simulink library "Local_Lib"  (R2023a)
settings: Solver=VariableStepAuto  StartTime=0.0  StopTime=10.0  RelTol=1e-3
settings Model: Creator=62555  LastModifiedBy=62555

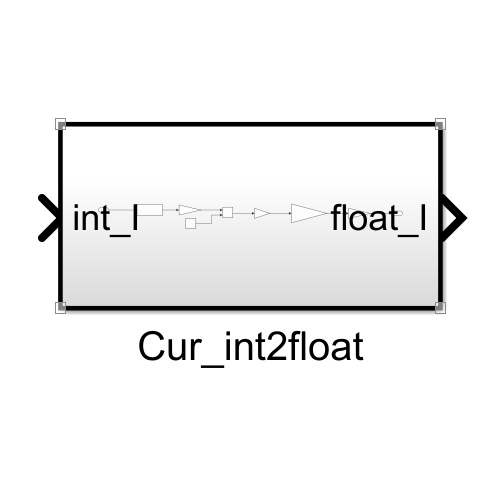
[thumbnail: Simulink's stored preview of the top-level diagram]
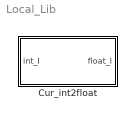
== system Local_Lib ==
  Cur_int2float : Subsystem  TreatAsAtomicUnit=on  RTWFileName=Local_Lib
      settings: RTWFcnNameOpts=Use subsystem name  RTWFileNameOpts=User specified

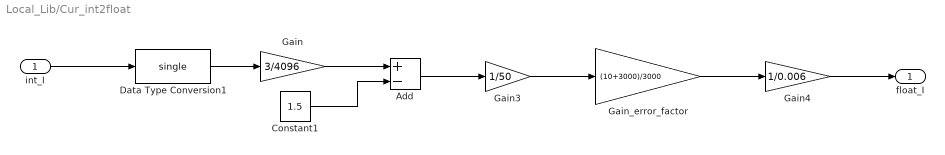
== system Local_Lib/Cur_int2float ==
  int_I : Inport
  Add : Sum  Inputs=+-
  Constant1 : Constant  Value=1.5  OutDataTypeStr=single  SampleTime=-1
  Data Type Conversion1 : DataTypeConversion  OutDataTypeStr=single  SaturateOnIntegerOverflow=off  RndMeth=Floor
  Gain : Gain  Gain=3/4096
  Gain3 : Gain  Gain=1/50
  Gain4 : Gain  Gain=1/0.006
  Gain_error_factor : Gain  Gain=(10+3000)/3000
  float_I : Outport
  wires:
  Add/1 -> Gain3/1
  Gain4/1 -> float_I/1
  Constant1/1 -> Add/2
  Gain/1 -> Add/1
  int_I/1 -> Data Type Conversion1/1
  Data Type Conversion1/1 -> Gain/1
  Gain3/1 -> Gain_error_factor/1
  Gain_error_factor/1 -> Gain4/1
